simulink model "2_2"  (R2021a)
settings: Solver=VariableStepAuto  StartTime=0.0  StopTime=1  RelTol=1e-3
values from neighbouring files (symbols this model uses):
  A = [2 6; 1 0]    [LR_10.m]
  B = [4; 1]    [LR_10.m]
  C = [2 0]    [LR_10.m]
  K = double([sol.k1(4) -sol.k2(4)])    [LR_10.m]
undefined symbols (not defined in the file or in its folder): F_h, L, M0
settings Model: Creator=fedor  LastModifiedBy=fedor

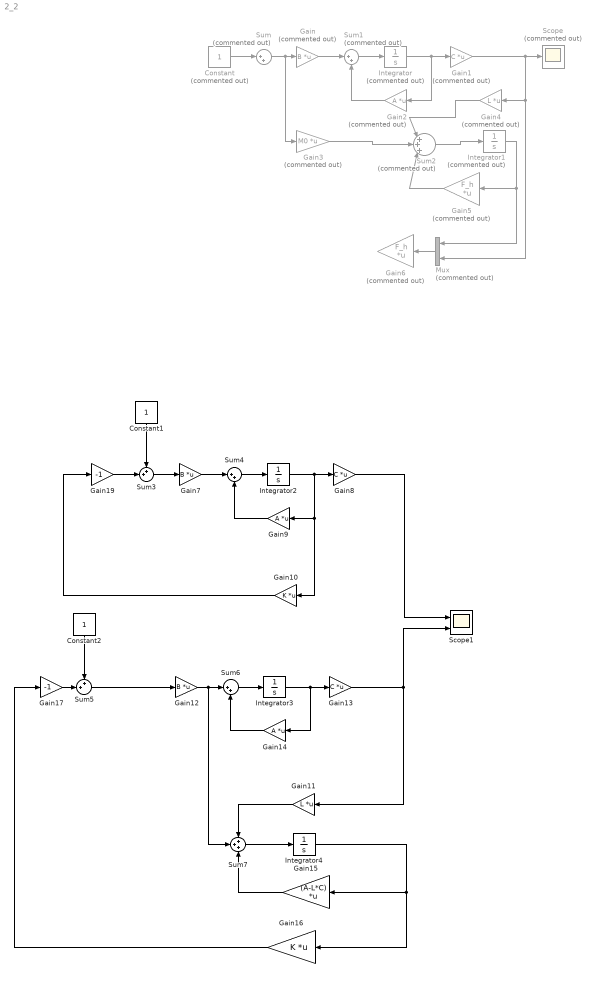
== system 2_2 ==
  Constant : Constant  Commented=on
  Constant1 : Constant
  Constant2 : Constant
  Gain : Gain  Commented=on  Gain=B  Multiplication=Matrix(K*u)
  Gain1 : Gain  Commented=on  Gain=C  Multiplication=Matrix(K*u)
  Gain10 : Gain  Gain=K  Multiplication=Matrix(K*u)
  Gain11 : Gain  Gain=L  Multiplication=Matrix(K*u)
  Gain12 : Gain  Gain=B  Multiplication=Matrix(K*u)
  Gain13 : Gain  Gain=C  Multiplication=Matrix(K*u)
  Gain14 : Gain  Gain=A  Multiplication=Matrix(K*u)
  Gain15 : Gain  Gain=(A-L*C)  Multiplication=Matrix(K*u)
  Gain16 : Gain  Gain=K  Multiplication=Matrix(K*u)
  Gain17 : Gain  Gain=-1
  Gain19 : Gain  Gain=-1
  Gain2 : Gain  Commented=on  Gain=A  Multiplication=Matrix(K*u)
  Gain3 : Gain  Commented=on  Gain=M0  Multiplication=Matrix(K*u)
  Gain4 : Gain  Commented=on  Gain=L  Multiplication=Matrix(K*u)
  Gain5 : Gain  Commented=on  Gain=F_h  Multiplication=Matrix(K*u)
  Gain6 : Gain  Commented=on  Gain=F_h  Multiplication=Matrix(K*u)
  Gain7 : Gain  Gain=B  Multiplication=Matrix(K*u)
  Gain8 : Gain  Gain=C  Multiplication=Matrix(K*u)
  Gain9 : Gain  Gain=A  Multiplication=Matrix(K*u)
  Integrator : Integrator  Commented=on
  Integrator1 : Integrator  Commented=on
  Integrator2 : Integrator
  Integrator3 : Integrator
  Integrator4 : Integrator
  Mux : Mux  Commented=on  Inputs=2
  Scope : Scope  Commented=on
  Scope1 : Scope  NumInputPorts=2
  Sum : Sum  Commented=on  Inputs=|++
  Sum1 : Sum  Commented=on  Inputs=|++
  Sum2 : Sum  Commented=on  Inputs=|+++|
  Sum3 : Sum  Inputs=++|
  Sum4 : Sum  Inputs=|++
  Sum5 : Sum  Inputs=++|
  Sum6 : Sum  Inputs=|++
  Sum7 : Sum  Inputs=+++
  wires:
  Constant/1 -> Sum/1
  Sum/1 -> Gain3/1, Gain/1
  Gain/1 -> Sum1/1
  Sum1/1 -> Integrator/1
  Integrator/1 -> Gain2/1, Gain1/1
  Gain2/1 -> Sum1/2
  Gain3/1 -> Sum2/2
  Gain4/1 -> Sum2/1
  Gain1/1 -> Gain4/1, Mux/2, Scope/1
  Sum2/1 -> Integrator1/1
  Gain5/1 -> Sum2/3
  Integrator1/1 -> Mux/1, Gain5/1
  Mux/1 -> Gain6/1
  Gain9/1 -> Sum4/2
  Integrator2/1 -> Gain10/1, Gain9/1, Gain8/1
  Gain7/1 -> Sum4/1
  Gain8/1 -> Scope1/1
  Sum4/1 -> Integrator2/1
  Sum3/1 -> Gain7/1
  Gain10/1 -> Gain19/1
  Constant1/1 -> Sum3/1
  Sum6/1 -> Integrator3/1
  Integrator3/1 -> Gain14/1, Gain13/1
  Gain12/1 -> Sum7/2, Sum6/1
  Gain14/1 -> Sum6/2
  Sum5/1 -> Gain12/1
  Constant2/1 -> Sum5/1
  Gain11/1 -> Sum7/1
  Sum7/1 -> Integrator4/1
  Integrator4/1 -> Gain15/1, Gain16/1
  Gain16/1 -> Gain17/1
  Gain17/1 -> Sum5/2
  Gain19/1 -> Sum3/2
  Gain13/1 -> Scope1/2, Gain11/1
  Gain15/1 -> Sum7/3
